simulink model "Linm_tf"  (Simulink 7.5)
settings: Solver=ode45  StartTime=0.0  StopTime=10.0  RelTol=1e-3
undefined symbols (not defined in the file): Chain
settings Model: Creator=fclaveau  LastModifiedBy=fclaveau

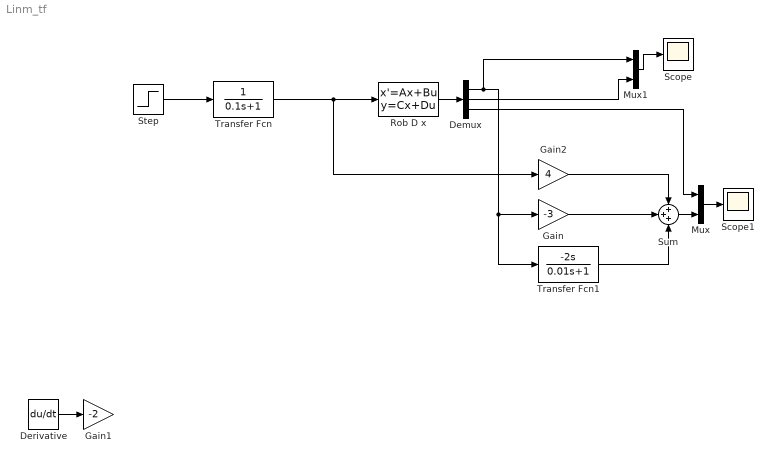
== system Linm_tf ==
  Demux : Demux  Outputs=3
  Derivative : Derivative
  Gain : Gain  Gain=-3  ParameterDataType=fixdt(1, 16)  ParameterScaling=2^0  OutDataType=fixdt(1, 16)  OutScaling=2^0
  Gain1 : Gain  Gain=-2  ParameterDataType=fixdt(1, 16)  ParameterScaling=2^0  OutDataType=fixdt(1, 16)  OutScaling=2^0
  Gain2 : Gain  Gain=4  ParameterDataType=fixdt(1, 16)  ParameterScaling=2^0  OutDataType=fixdt(1, 16)  OutScaling=2^0
  Mux : Mux  Inputs=2
  Mux1 : Mux  Inputs=2
  "Rob D x " : StateSpace  A=Chain.A  B=Chain.B  C=Chain.C  D=Chain.D
  Scope : Scope
  Scope1 : Scope
  Step : Step  SampleTime=0
  Sum : Sum  Inputs=+++  OutDataType=fixdt(1, 16)  OutScaling=2^0
  Transfer Fcn : TransferFcn  Denominator=[0.1 1]
  Transfer Fcn1 : TransferFcn  Numerator=[-2 0]  Denominator=[0.01 1]
  wires:
  "Rob D x "/1 -> Demux/1
  Step/1 -> Transfer Fcn/1
  Demux/1 -> Gain/1, Transfer Fcn1/1, Mux1/1
  Mux/1 -> Scope1/1
  Sum/1 -> Mux/2
  Demux/3 -> Mux/1
  Mux1/1 -> Scope/1
  Demux/2 -> Mux1/2
  Gain2/1 -> Sum/1
  Gain/1 -> Sum/2
  Transfer Fcn1/1 -> Sum/3
  Transfer Fcn/1 -> "Rob D x "/1, Gain2/1
  Derivative/1 -> Gain1/1
